simulink model "dual_motor"  (R2020a)
settings: Solver=FixedStepDiscrete  StartTime=0.0  StopTime=10.0  RelTol=1e-3  EnableMultiTasking=on
libraries: REG_Lib x6, TIMERS_Lib x5, GPIO_Lib x3, simulink x2, STM32_Config_Lib x1, USART_Lib x1
settings Model: Creator=Gang  LastModifiedBy=tuziz
settings DataIOCC: LimitDataPoints=on  SaveFormat=Array  ReturnWorkspaceOutputs=off
settings OptimizationCC: DefaultParameterBehavior=Inlined  DefaultUnderspecifiedDataType=single  LifeSpan=1  EfficientTunableParamExpr=on
settings DebuggingCC: UnderspecifiedInitializationDetection=Classic  MergeDetectMultiDrivingBlocksExec=none  InheritedTsInSrcMsg=none  UniqueDataStoreMsg=error  AllowSymbolicDim=off  StrictBusMsg=ErrorOnBusTreatedAsVector  SFUnexpectedBacktrackingDiag=warning  SFNoUnconditionalDefaultTransitionDiag=warning  SFUndirectedBroadcastEventsDiag=error  SFExecutionAtInitializationDiag=none  ArithmeticOperatorsInVariantConditions=warning
settings HardwareCC: ProdBitPerPointer=32  ProdBitPerSizeT=32  ProdBitPerPtrDiffT=32  ProdLargestAtomicInteger=Integer  ProdWordSize=32  ProdHWDeviceType=STMicroelectronics->STM32 32-bit Cortex-M
settings ModelReferenceCC: PropagateSignalLabelsOutOfModel=off
settings SFSimCC: SimUseLocalCustomCode=off  CompileTimeRecursionLimit=0  EnableRuntimeRecursion=off  MATLABDynamicMemAlloc=off  CustomCodeUndefinedFunction=UseInterfaceOnly
settings RTWCC: Description=stm32 (Embedded Target)  SystemTargetFile=stm32.tlc  TemplateMakefile=stm32.tmf  GenerateReport=on  RTWUseLocalCustomCode=off
settings CodeAppCC: IgnoreCustomStorageClasses=off  CustomSymbolStrType=$N$R$M  SimulinkBlockComments=off
settings STFCustomTargetCC: TargetLangStandard=C99 (ISO)  ParMdlRefBuildCompliant=on  IncludeMdlTerminateFcn=off  CombineOutputUpdateFcns=on  ERTCustomFileBanners=on  SupportComplex=off  SupportContinuousTime=off  SupportNonInlinedSFcns=off  RemoveResetFunc=on  ParenthesesLevel=Maximum  CastingMode=Standards  MATLABClassNameForMDSCustomization=Simulink.SoftwareTarget.ERTCustomization  SystemTargetFile=stm32.tlc
settings ERTTargetCC: TargetLangStandard=C99 (ISO)  MultiwordLength=2048  CompOptLevelCompliant=off  ConcurrentExecutionCompliant=off  IncludeMdlTerminateFcn=off  SupportComplex=off  ParenthesesLevel=Maximum  CastingMode=Standards  ModelStepFunctionPrototypeControlCompliant=off  CPPClassGenCompliant=off  UseToolchainInfoCompliant=off  ERTSrcFileBannerTemplate=sourceFileTemplate.cgt  ERTHdrFileBannerTemplate=sourceFileTemplate.cgt  ERTDataSrcFileTemplate=sourceFileTemplate.cgt  ERTDataHdrFileTemplate=sourceFileTemplate.cgt  ERTCustomFileTemplate=customRoutineProcess.tlc  ConvertIfToSwitch=off  SuppressUnreachableDefaultCases=off  EnableSignedLeftShifts=off  EnableSignedRightShifts=off
settings ConfigComp: CovMetricSettings=dw  CovHtmlReporting=on  CovSaveCumulativeToWorkspaceVar=on  CovSaveSingleToWorkspaceVar=on  CovExternalEMLEnable=off  CovSFcnEnable=off

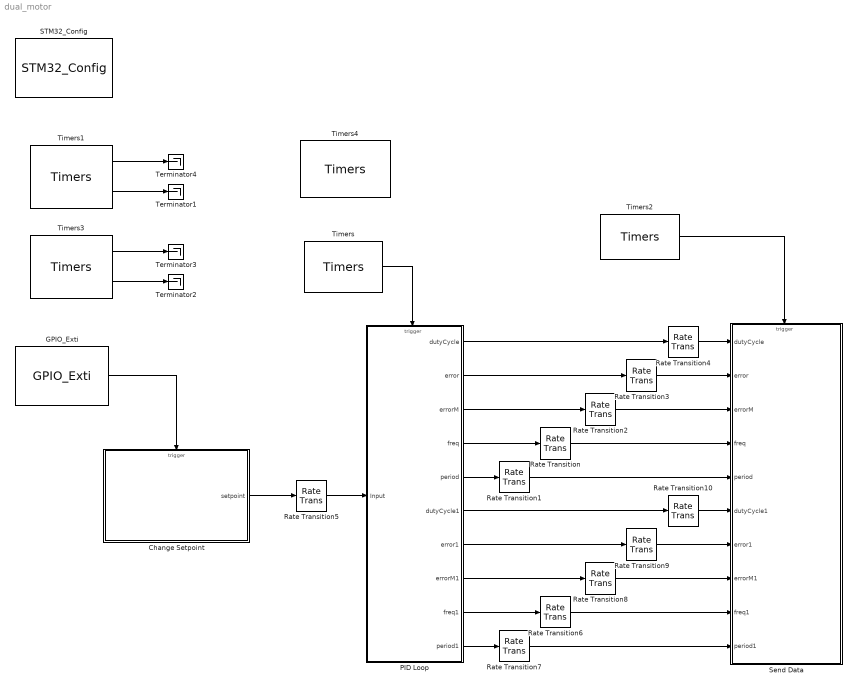
== system dual_motor ==
  Change Setpoint : Subsystem  TreatAsAtomicUnit=on
  GPIO_Exti : GPIO_Lib/GPIO_Exti  Port_name=GPIOA  Pin_0=on  Pin_1=off  Pin_2=off  Pin_3=off  Pin_4=off  Pin_5=off  Pin_6=off  Pin_7=off  Pin_8=off  Pin_9=off  Pin_10=off  Pin_11=off  Pin_12=off  Pin_13=off  Pin_14=off  Pin_15=off  PinList=GPIOA0
      settings: SourceProductName=Target Support Package - STM32 Adapter
  PID Loop : Subsystem  TreatAsAtomicUnit=on
  Rate Transition{,1..10} (11 alike) : RateTransition  Deterministic=off
  STM32_Config : STM32_Config_Lib/STM32_Config  Priority=0  Project_Path=.\  Config_File=dual_motor.ioc  MCU_Name=STM32F407VGTx
      settings: SourceProductName=Target Support Package - STM32 Adapter
  Send Data : Subsystem  TreatAsAtomicUnit=on
  Terminator{1..4} (4 alike) : Terminator
  Timers : TIMERS_Lib/Timers  currentTIM=TIM6  TIM_Name=TIM6  sysUsingTimer=off  TIM_APBClock=84000000  TIM_Set_Clk=off  TIM_Prescaler=8400-1  TIM_Clock=10000.00  Variable_frequency=off  TIM_Set_OutFreq=off  TIM_ARR=10  Output_frequency=1000.00  Repetition_counter=0  TIM_Mode=Up  TIM_DMA=none  TIM_IRQ=off  TIM_IRQ_ONLY=on  TIM_UP=on  TIM_TRG=off  TIM_COM=off  TIM_BRK=off  NbTIM=5  CH1_enable=off  CH1N_enable=off  CH1_type=Unknown  CH1_DMA=off  CH1_int=off  CH1_edge=Rising  CH1_div=1  CH1_variable_duty=off  CH1_set_pulse=off  CH1_output_duty=0.00  CH1_pulse=0  CH2_enable=off  CH2N_enable=off  CH2_type=Unknown  CH2_DMA=off  CH2_int=off  CH2_edge=Rising  CH2_div=1  CH2_variable_duty=off  CH2_set_pulse=off  CH2_output_duty=0.00  CH2_pulse=0  CH3_enable=off  CH3N_enable=off  CH3_type=Unknown  CH3_DMA=off  CH3_int=off  CH3_edge=Rising  CH3_div=1  CH3_variable_duty=off  CH3_set_pulse=off  CH3_output_duty=0.00  CH3_pulse=0  CH4_enable=off  CH4N_enable=off  CH4_type=Unknown  CH4_DMA=off  CH4_int=off  CH4_edge=Rising  CH4_div=1  CH4_variable_duty=off  CH4_set_pulse=off  CH4_output_duty=0.00  CH4_pulse=0
      settings: SourceProductName=Target Support Package - STM32 Adapter
  Timers1 : TIMERS_Lib/Timers  currentTIM=TIM3  TIM_Name=TIM3  sysUsingTimer=off  TIM_APBClock=84000000  TIM_Set_Clk=off  TIM_Prescaler=840-1  TIM_Clock=100000.00  Variable_frequency=off  TIM_Set_OutFreq=off  TIM_ARR=2000  Output_frequency=50.00  Repetition_counter=0  TIM_Mode=Up  TIM_DMA=none  TIM_IRQ=off  TIM_IRQ_ONLY=off  TIM_UP=off  TIM_TRG=off  TIM_COM=off  TIM_BRK=off  NbTIM=5  CH1_enable=on  CH1N_enable=off  CH1_type=Input_Capture  CH1_DMA=off  CH1_int=on  CH1_edge=Rising  CH1_div=1  CH1_variable_duty=off  CH1_set_pulse=off  CH1_output_duty=0.00  CH1_pulse=0  CH2_enable=off  CH2N_enable=off  CH2_type=Input_Capture  CH2_DMA=off  CH2_int=off  CH2_edge=Rising  CH2_div=1  CH2_variable_duty=off  CH2_set_pulse=off  CH2_output_duty=0.00  CH2_pulse=0  CH3_enable=off  CH3N_enable=off  CH3_type=Unknown  CH3_DMA=off  CH3_int=off  CH3_edge=Rising  CH3_div=1  CH3_variable_duty=off  CH3_set_pulse=off  CH3_output_duty=0.00  CH3_pulse=0  CH4_enable=off  CH4N_enable=off  CH4_type=Unknown  CH4_DMA=off  CH4_int=off  CH4_edge=Rising  CH4_div=1  CH4_variable_duty=off  CH4_set_pulse=off  CH4_output_duty=0.00  CH4_pulse=0
      settings: SourceProductName=Target Support Package - STM32 Adapter
  Timers2 : TIMERS_Lib/Timers  currentTIM=TIM7  TIM_Name=TIM7  sysUsingTimer=off  TIM_APBClock=84000000  TIM_Set_Clk=off  TIM_Prescaler=840-1  TIM_Clock=100000.00  Variable_frequency=off  TIM_Set_OutFreq=off  TIM_ARR=1000  Output_frequency=100.00  Repetition_counter=0  TIM_Mode=Up  TIM_DMA=none  TIM_IRQ=off  TIM_IRQ_ONLY=on  TIM_UP=on  TIM_TRG=off  TIM_COM=off  TIM_BRK=off  NbTIM=5  CH1_enable=off  CH1N_enable=off  CH1_type=Unknown  CH1_DMA=off  CH1_int=off  CH1_edge=Rising  CH1_div=1  CH1_variable_duty=off  CH1_set_pulse=off  CH1_output_duty=0.00  CH1_pulse=0  CH2_enable=off  CH2N_enable=off  CH2_type=Unknown  CH2_DMA=off  CH2_int=off  CH2_edge=Rising  CH2_div=1  CH2_variable_duty=off  CH2_set_pulse=off  CH2_output_duty=0.00  CH2_pulse=0  CH3_enable=off  CH3N_enable=off  CH3_type=Unknown  CH3_DMA=off  CH3_int=off  CH3_edge=Rising  CH3_div=1  CH3_variable_duty=off  CH3_set_pulse=off  CH3_output_duty=0.00  CH3_pulse=0  CH4_enable=off  CH4N_enable=off  CH4_type=Unknown  CH4_DMA=off  CH4_int=off  CH4_edge=Rising  CH4_div=1  CH4_variable_duty=off  CH4_set_pulse=off  CH4_output_duty=0.00  CH4_pulse=0
      settings: SourceProductName=Target Support Package - STM32 Adapter
  Timers3 : TIMERS_Lib/Timers  currentTIM=TIM4  TIM_Name=TIM4  sysUsingTimer=off  TIM_APBClock=84000000  TIM_Set_Clk=off  TIM_Prescaler=840-1  TIM_Clock=100000.00  Variable_frequency=off  TIM_Set_OutFreq=off  TIM_ARR=2000  Output_frequency=50.00  Repetition_counter=0  TIM_Mode=Up  TIM_DMA=none  TIM_IRQ=off  TIM_IRQ_ONLY=off  TIM_UP=off  TIM_TRG=off  TIM_COM=off  TIM_BRK=off  NbTIM=5  CH1_enable=on  CH1N_enable=off  CH1_type=Input_Capture  CH1_DMA=off  CH1_int=on  CH1_edge=Rising  CH1_div=1  CH1_variable_duty=off  CH1_set_pulse=off  CH1_output_duty=0.00  CH1_pulse=0  CH2_enable=off  CH2N_enable=off  CH2_type=Unknown  CH2_DMA=off  CH2_int=off  CH2_edge=Rising  CH2_div=1  CH2_variable_duty=off  CH2_set_pulse=off  CH2_output_duty=0.00  CH2_pulse=0  CH3_enable=off  CH3N_enable=off  CH3_type=Unknown  CH3_DMA=off  CH3_int=off  CH3_edge=Rising  CH3_div=1  CH3_variable_duty=off  CH3_set_pulse=off  CH3_output_duty=0.00  CH3_pulse=0  CH4_enable=off  CH4N_enable=off  CH4_type=Unknown  CH4_DMA=off  CH4_int=off  CH4_edge=Rising  CH4_div=1  CH4_variable_duty=off  CH4_set_pulse=off  CH4_output_duty=0.00  CH4_pulse=0
      settings: SourceProductName=Target Support Package - STM32 Adapter
  Timers4 : TIMERS_Lib/Timers  currentTIM=TIM9  TIM_Name=TIM9  sysUsingTimer=off  TIM_APBClock=168000000  TIM_Set_Clk=off  TIM_Prescaler=3359  TIM_Clock=50000.00  Variable_frequency=off  TIM_Set_OutFreq=off  TIM_ARR=100  Output_frequency=500.00  Repetition_counter=0  TIM_Mode=Up  TIM_DMA=none  TIM_IRQ=off  TIM_IRQ_ONLY=off  TIM_UP=off  TIM_TRG=off  TIM_COM=off  TIM_BRK=off  NbTIM=5  CH1_enable=on  CH1N_enable=off  CH1_type=Output_PWM  CH1_DMA=off  CH1_int=off  CH1_edge=Rising  CH1_div=1  CH1_variable_duty=off  CH1_set_pulse=off  CH1_output_duty=0.00  CH1_pulse=0  CH2_enable=on  CH2N_enable=off  CH2_type=Output_PWM  CH2_DMA=off  CH2_int=off  CH2_edge=Rising  CH2_div=1  CH2_variable_duty=off  CH2_set_pulse=off  CH2_output_duty=0.00  CH2_pulse=0  CH3_enable=off  CH3N_enable=off  CH3_type=Unknown  CH3_DMA=off  CH3_int=off  CH3_edge=Rising  CH3_div=1  CH3_variable_duty=off  CH3_set_pulse=off  CH3_output_duty=0.00  CH3_pulse=0  CH4_enable=off  CH4N_enable=off  CH4_type=Unknown  CH4_DMA=off  CH4_int=off  CH4_edge=Rising  CH4_div=1  CH4_variable_duty=off  CH4_set_pulse=off  CH4_output_duty=0.00  CH4_pulse=0
      settings: SourceProductName=Target Support Package - STM32 Adapter
  wires:
  Timers2/1 -> Send Data/Trigger
  Timers1/2 -> Terminator1/1
  PID Loop/4(freq) -> Rate Transition/1
  PID Loop/5(period) -> Rate Transition1/1
  Rate Transition/1 -> Send Data/4(freq)
  Rate Transition1/1 -> Send Data/5(period)
  Rate Transition2/1 -> Send Data/3(errorM)
  PID Loop/3(errorM) -> Rate Transition2/1
  PID Loop/2(error) -> Rate Transition3/1
  Rate Transition3/1 -> Send Data/2(error)
  Rate Transition4/1 -> Send Data/1(dutyCycle)
  PID Loop/1(dutyCycle) -> Rate Transition4/1
  GPIO_Exti/1 -> Change Setpoint/Trigger
  Change Setpoint/1(setpoint) -> Rate Transition5/1
  Rate Transition5/1 -> PID Loop/1(Input)
  PID Loop/6(dutyCycle1) -> Rate Transition10/1
  Rate Transition9/1 -> Send Data/7(error1)
  PID Loop/7(error1) -> Rate Transition9/1
  PID Loop/8(errorM1) -> Rate Transition8/1
  Rate Transition8/1 -> Send Data/8(errorM1)
  Rate Transition7/1 -> Send Data/10(period1)
  Rate Transition6/1 -> Send Data/9(freq1)
  PID Loop/9(freq1) -> Rate Transition6/1
  PID Loop/10(period1) -> Rate Transition7/1
  Rate Transition10/1 -> Send Data/6(dutyCycle1)
  Timers3/1 -> Terminator3/1
  Timers3/2 -> Terminator2/1
  Timers1/1 -> Terminator4/1
  Timers/1 -> PID Loop/Trigger

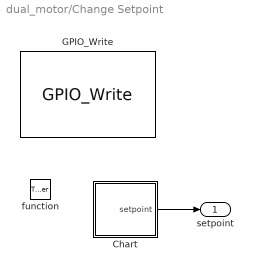
== system dual_motor/Change Setpoint ==
  function : TriggerPort  TriggerType=function-call  VariantControl=Variant  OutputDataType=int8
  Chart : Stateflow chart  TreatAsAtomicUnit=on
  GPIO_Write : GPIO_Lib/GPIO_Write  Port_name=GPIOD  Pin0=off  Toggle_Pin0=off  Pin1=off  Toggle_Pin1=off  Pin2=off  Toggle_Pin2=off  Pin3=off  Toggle_Pin3=off  Pin4=off  Toggle_Pin4=off  Pin5=off  Toggle_Pin5=off  Pin6=off  Toggle_Pin6=off  Pin7=off  Toggle_Pin7=off  Pin8=off  Toggle_Pin8=off  Pin9=off  Toggle_Pin9=off  Pin10=off  Toggle_Pin10=off  Pin11=off  Toggle_Pin11=off  Pin12=off  Toggle_Pin12=off  Pin13=off  Toggle_Pin13=off  Pin14=on  Toggle_Pin14=on  Pin15=off  Toggle_Pin15=off  PinList="GPIOD12  13  14  15"
      settings: SourceProductName=Target Support Package - STM32 Adapter
  setpoint : Outport
  wires:
  Chart/1(setpoint) -> setpoint/1

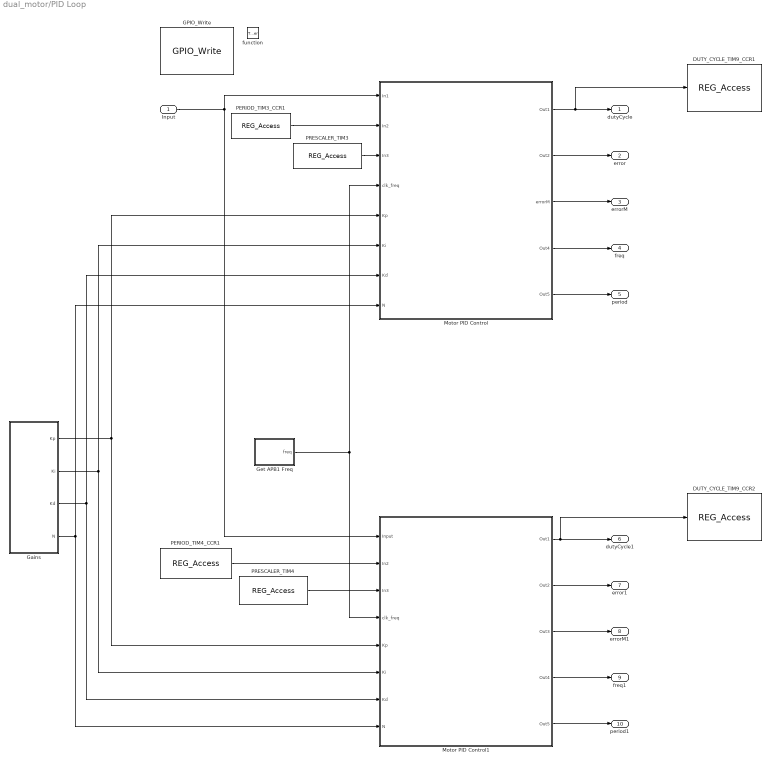
== system dual_motor/PID Loop ==
  Input : Inport
  function : TriggerPort  TriggerType=function-call  VariantControl=Variant
  DUTY_CYCLE_TIM9_CCR1 : REG_Lib/REG_Access  Peripheral=TIM9  RegName=CCR1  RegRead=off  RegWrite=on  RegValueIn=on  RegEqual=on  RegAnd=off  RegOr=off  RegComplement=off  currentPeriph=TIM9
      settings: SourceProductName=Target Support Package - STM32 Adapter
  DUTY_CYCLE_TIM9_CCR2 : REG_Lib/REG_Access  Peripheral=TIM9  RegName=CCR2  RegRead=off  RegWrite=on  RegValueIn=on  RegEqual=on  RegAnd=off  RegOr=off  RegComplement=off  currentPeriph=TIM9
      settings: SourceProductName=Target Support Package - STM32 Adapter
  GPIO_Write : GPIO_Lib/GPIO_Write  Port_name=GPIOD  Pin0=off  Toggle_Pin0=off  Pin1=off  Toggle_Pin1=off  Pin2=off  Toggle_Pin2=off  Pin3=off  Toggle_Pin3=off  Pin4=off  Toggle_Pin4=off  Pin5=off  Toggle_Pin5=off  Pin6=off  Toggle_Pin6=off  Pin7=off  Toggle_Pin7=off  Pin8=off  Toggle_Pin8=off  Pin9=off  Toggle_Pin9=off  Pin10=off  Toggle_Pin10=off  Pin11=off  Toggle_Pin11=off  Pin12=off  Toggle_Pin12=off  Pin13=on  Toggle_Pin13=on  Pin14=off  Toggle_Pin14=off  Pin15=off  Toggle_Pin15=off  PinList="GPIOD12  13  14  15"
      settings: SourceProductName=Target Support Package - STM32 Adapter
  Gains : MATLAB Function  TreatAsAtomicUnit=on
  Get APB1 Freq : MATLAB Function  TreatAsAtomicUnit=on
  Motor PID Control : Subsystem
  Motor PID Control1 : Subsystem
  PERIOD_TIM3_CCR1 : REG_Lib/REG_Access  Peripheral=TIM3  RegName=CCR1  RegRead=on  RegWrite=off  RegValueIn=off  RegEqual=on  RegAnd=off  RegOr=off  RegComplement=off  currentPeriph=TIM3
      settings: SourceProductName=Target Support Package - STM32 Adapter
  PERIOD_TIM4_CCR1 : REG_Lib/REG_Access  Peripheral=TIM4  RegName=CCR1  RegRead=on  RegWrite=off  RegValueIn=off  RegEqual=on  RegAnd=off  RegOr=off  RegComplement=off  currentPeriph=TIM4
      settings: SourceProductName=Target Support Package - STM32 Adapter
  PRESCALER_TIM3 : REG_Lib/REG_Access  Peripheral=TIM3  RegName=PSC  RegRead=on  RegWrite=off  RegValueIn=off  RegEqual=on  RegAnd=off  RegOr=off  RegComplement=off  currentPeriph=TIM3
      settings: SourceProductName=Target Support Package - STM32 Adapter
  PRESCALER_TIM4 : REG_Lib/REG_Access  Peripheral=TIM4  RegName=PSC  RegRead=on  RegWrite=off  RegValueIn=off  RegEqual=on  RegAnd=off  RegOr=off  RegComplement=off  currentPeriph=TIM4
      settings: SourceProductName=Target Support Package - STM32 Adapter
  dutyCycle : Outport
  error : Outport  Port=2
  errorM : Outport  Port=3
  freq : Outport  Port=4
  period : Outport  Port=5
  dutyCycle1 : Outport  Port=6
  error1 : Outport  Port=7
  errorM1 : Outport  Port=8
  freq1 : Outport  Port=9
  period1 : Outport  Port=10
  wires:
  Motor PID Control/1(Out1) -> DUTY_CYCLE_TIM9_CCR1/1, dutyCycle/1
  PERIOD_TIM3_CCR1/1 -> Motor PID Control/2(In2)
  Motor PID Control/2(Out2) -> error/1
  Motor PID Control/4(Out4) -> freq/1
  Motor PID Control/5(Out5) -> period/1
  Input/1 -> Motor PID Control1/1(Input), Motor PID Control/1(In1)
  Motor PID Control1/5(Out5) -> period1/1
  Motor PID Control1/4(Out4) -> freq1/1
  Motor PID Control1/3(Out3) -> errorM1/1
  Motor PID Control1/2(Out2) -> error1/1
  PERIOD_TIM4_CCR1/1 -> Motor PID Control1/2(In2)
  Motor PID Control1/1(Out1) -> DUTY_CYCLE_TIM9_CCR2/1, dutyCycle1/1
  Get APB1 Freq/1(freq) -> Motor PID Control/4(clk_freq), Motor PID Control1/4(clk_freq)
  PRESCALER_TIM3/1 -> Motor PID Control/3(In3)
  PRESCALER_TIM4/1 -> Motor PID Control1/3(In3)
  Motor PID Control/3(errorM) -> errorM/1
  Gains/1(Kp) -> Motor PID Control/5(Kp), Motor PID Control1/5(Kp)
  Gains/2(Ki) -> Motor PID Control/6(Ki), Motor PID Control1/6(Ki)
  Gains/3(Kd) -> Motor PID Control/7(Kd), Motor PID Control1/7(Kd)
  Gains/4(N) -> Motor PID Control/8(N), Motor PID Control1/8(N)

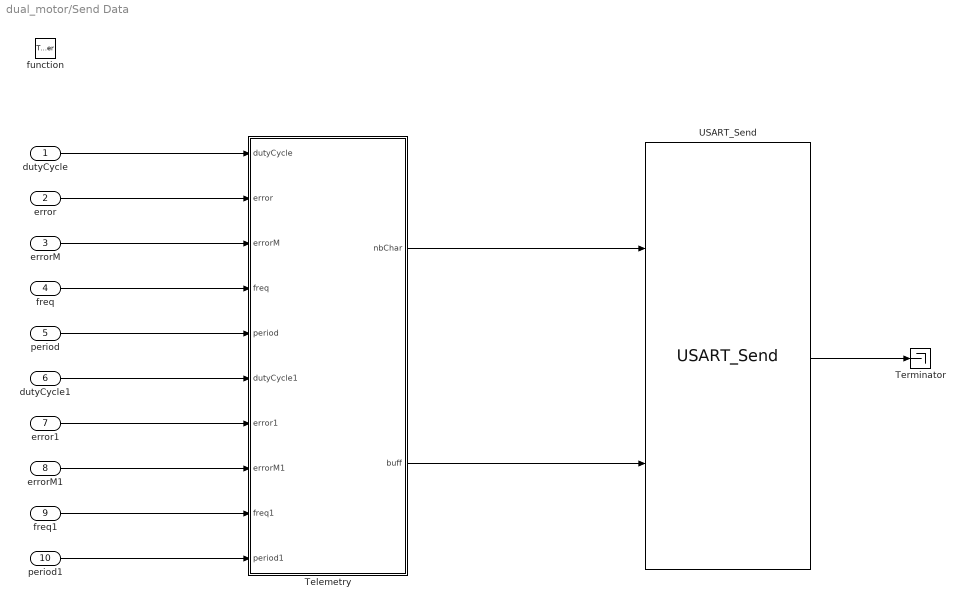
== system dual_motor/Send Data ==
  dutyCycle : Inport
  error : Inport  Port=2
  errorM : Inport  Port=3
  freq : Inport  Port=4
  period : Inport  Port=5
  dutyCycle1 : Inport  Port=6
  error1 : Inport  Port=7
  errorM1 : Inport  Port=8
  freq1 : Inport  Port=9
  period1 : Inport  Port=10
  function : TriggerPort  TriggerType=function-call  VariantControl=Variant
  Telemetry : MATLAB Function  TreatAsAtomicUnit=on
  Terminator : Terminator
  USART_Send : USART_Lib/USART_Send  USART_name=USART3  Buff_size=512  nbUsart=1  usartMode=Asynchronous  usartDma_Rx=off  usartDma_Tx=off  usartIt=off
      settings: SourceProductName=Target Support Package - STM32 Adapter
  wires:
  USART_Send/1 -> Terminator/1
  period/1 -> Telemetry/5(period)
  freq/1 -> Telemetry/4(freq)
  dutyCycle/1 -> Telemetry/1(dutyCycle)
  error/1 -> Telemetry/2(error)
  errorM/1 -> Telemetry/3(errorM)
  Telemetry/1(nbChar) -> USART_Send/1
  Telemetry/2(buff) -> USART_Send/2
  period1/1 -> Telemetry/10(period1)
  freq1/1 -> Telemetry/9(freq1)
  dutyCycle1/1 -> Telemetry/6(dutyCycle1)
  error1/1 -> Telemetry/7(error1)
  errorM1/1 -> Telemetry/8(errorM1)

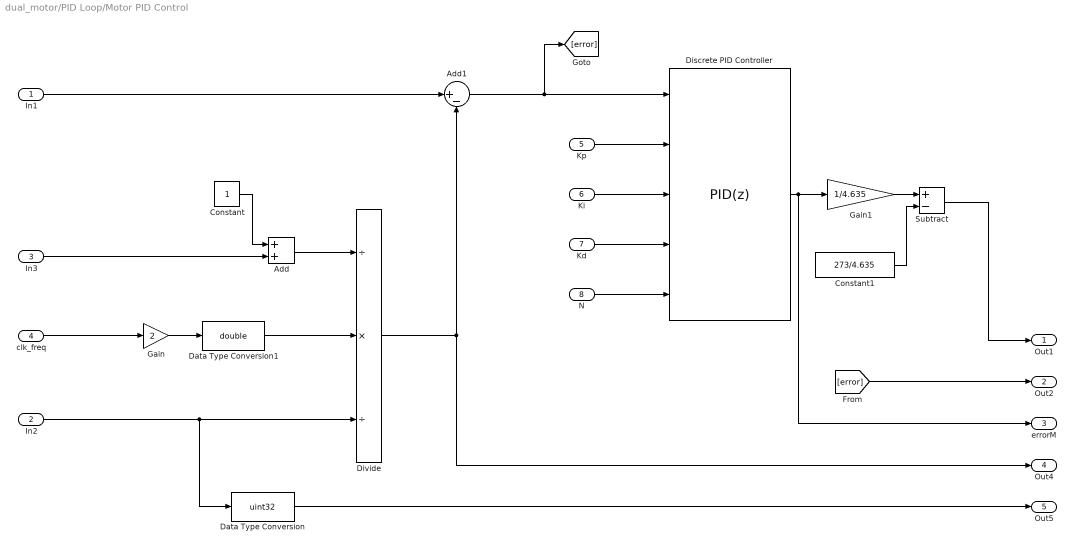
== system dual_motor/PID Loop/Motor PID Control ==
  In1 : Inport
  In2 : Inport  Port=2
  In3 : Inport  Port=3
  clk_freq : Inport  Port=4
  Kp : Inport  Port=5
  Ki : Inport  Port=6
  Kd : Inport  Port=7
  N : Inport  Port=8
  Add : Sum  OutDataTypeStr=double
  Add1 : Sum  Inputs=|+-  OutDataTypeStr=double
  Constant : Constant  OutDataTypeStr=double
  Constant1 : Constant  Value=273/4.635
  Data Type Conversion : DataTypeConversion  OutDataTypeStr=uint32
  Data Type Conversion1 : DataTypeConversion  OutDataTypeStr=double
  Discrete PID Controller : simulink/Continuous/PID Controller  Controller=PID  Form=Parallel  TimeDomain=Discrete-time  UseExternalTs=off  SampleTime=-1  IntegratorMethod=Forward Euler  FilterMethod=Forward Euler  ControllerParametersSource=external  P=50.0  I=5  D=.5  UseFilter=on  N=100  TunerSelectOption=Transfer Function Based (PID Tuner App)  InitialConditionSource=internal  InitialConditionForIntegrator=0  InitialConditionForFilter=0  DifferentiatorICPrevScaledInput=0  ExternalReset=none  TrackingMode=off  Kt=1  LimitOutput=on  UpperSaturationLimit=700  LowerSaturationLimit=273  LinearizeAsGain=off  AntiWindupMode=clamping  Kb=1  POutMin=[]  POutMax=[]  IOutMin=[]  IOutMax=[]  DOutMin=[]  DOutMax=[]  NOutMin=[]  NOutMax=[]  SumOutMin=[]  SumOutMax=[]  SaturationOutMin=[]  SaturationOutMax=[]  PParamMin=[]  PParamMax=[]  IParamMin=[]  IParamMax=[]  DParamMin=[]  DParamMax=[]  NParamMin=[]  NParamMax=[]  KbParamMin=[]  KbParamMax=[]  KtParamMin=[]  KtParamMax=[]  KbOutMin=[]  KbOutMax=[]  KtOutMin=[]  KtOutMax=[]  IntegratorOutMin=[]  IntegratorOutMax=[]  FilterOutMin=[]  FilterOutMax=[]  SumI1OutMin=[]  SumI1OutMax=[]  SumI2OutMin=[]  SumI2OutMax=[]  SumI3OutMin=[]  SumI3OutMax=[]  SumI4OutMin=[]  SumI4OutMax=[]  SumDOutMin=[]  SumDOutMax=[]  DifferentiatorOutMin=[]  DifferentiatorOutMax=[]  FilterDiffOutCoefMin=[]  FilterDiffOutCoefMax=[]  ReciprocalOutMin=[]  ReciprocalOutMax=[]  SumDenOutMin=[]  SumDenOutMax=[]  SumNumOutMin=[]  SumNumOutMax=[]  DivideOutMin=[]  DivideOutMax=[]  UdiffTsProdOutMin=[]  UdiffTsProdOutMax=[]  NTsProdOutMin=[]  NTsProdOutMax=[]  UintegralTsProdOutMin=[]  UintegralTsProdOutMax=[]  UngainTsProdOutMin=[]  UngainTsProdOutMax=[]  IntegratorContinuousStateAttributes=''  IntegratorStateMustResolveToSignalObject=off  IntegratorRTWStateStorageClass=Auto  FilterContinuousStateAttributes=''  FilterStateMustResolveToSignalObject=off  FilterRTWStateStorageClass=Auto  ParallelPVariant=ExternalParameters  IdealPVariant=Disabled  IVariant=ExternalParameters  DVariant=ExternalParameters  IntegratorVariant=Discrete  SatVariant=Enabled  AWVariant=DiscClampingParallel  PCopyVariant=Disabled  TRVariant=Disabled  FdbkBlocksVariant=Forward  IdealPFdbkVariant=Disabled  SatFdbkVariant=Disabled  DerivativeFilterVariant=ForwardEulerFilter  NVariant=ExternalParameters  NCopyVariant=Disabled  FilterICVariant=InternalICsFilter  IntegratorICVariant=InternalICs  ExternalResetVariant=Disabled  TRSumVariant=Passthrough  SumFdbkVariant=Disabled  SumVariant=Sum_PID  TsampFilterVariant=InternalTs  TsampNgainVariant=Passthrough  TsampIntegralVariant=Passthrough
  Divide : Product  Inputs=/*/  OutDataTypeStr=double
  Gain : Gain  Gain=2  ParamDataTypeStr=double  OutDataTypeStr=double
  Gain1 : Gain  Gain=1/4.635  OutDataTypeStr=double
  Subtract : Sum  Inputs=+-
  Out1 : Outport
  Out2 : Outport  Port=2
  errorM : Outport  Port=3
  Out4 : Outport  Port=4
  Out5 : Outport  Port=5
  wires:
  In3/1 -> Add/2
  Data Type Conversion/1 -> Out5/1
  Add1/1 -> [error], Discrete PID Controller/1
  Constant/1 -> Add/1
  In2/1 -> Data Type Conversion/1, Divide/3
  Add/1 -> Divide/1
  Divide/1 -> Out4/1, Add1/2
  Discrete PID Controller/1 -> Gain1/1, errorM/1
  Kd/1 -> Discrete PID Controller/4
  clk_freq/1 -> Gain/1
  Kp/1 -> Discrete PID Controller/2
  Gain/1 -> Data Type Conversion1/1
  Ki/1 -> Discrete PID Controller/3
  [error] -> Out2/1
  Data Type Conversion1/1 -> Divide/2
  N/1 -> Discrete PID Controller/5
  In1/1 -> Add1/1
  Gain1/1 -> Subtract/1
  Subtract/1 -> Out1/1
  Constant1/1 -> Subtract/2

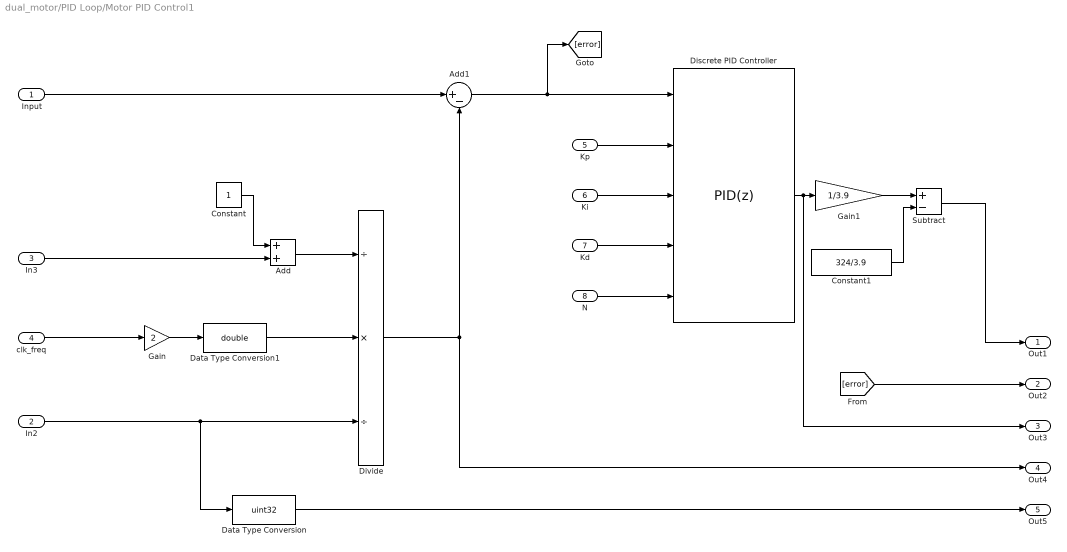
== system dual_motor/PID Loop/Motor PID Control1 ==
  Input : Inport
  In2 : Inport  Port=2
  In3 : Inport  Port=3
  clk_freq : Inport  Port=4
  Kp : Inport  Port=5
  Ki : Inport  Port=6
  Kd : Inport  Port=7
  N : Inport  Port=8
  Add : Sum  OutDataTypeStr=double
  Add1 : Sum  Inputs=|+-  OutDataTypeStr=double
  Constant : Constant  OutDataTypeStr=double
  Constant1 : Constant  Value=324/3.9
  Data Type Conversion : DataTypeConversion  OutDataTypeStr=uint32
  Data Type Conversion1 : DataTypeConversion  OutDataTypeStr=double
  Discrete PID Controller : simulink/Continuous/PID Controller  Controller=PID  Form=Parallel  TimeDomain=Discrete-time  UseExternalTs=off  SampleTime=-1  IntegratorMethod=Forward Euler  FilterMethod=Forward Euler  ControllerParametersSource=external  P=50.0  I=5  D=.5  UseFilter=on  N=100  TunerSelectOption=Transfer Function Based (PID Tuner App)  InitialConditionSource=internal  InitialConditionForIntegrator=0  InitialConditionForFilter=0  DifferentiatorICPrevScaledInput=0  ExternalReset=none  TrackingMode=off  Kt=1  LimitOutput=on  UpperSaturationLimit=700  LowerSaturationLimit=324  LinearizeAsGain=off  AntiWindupMode=clamping  Kb=1  POutMin=[]  POutMax=[]  IOutMin=[]  IOutMax=[]  DOutMin=[]  DOutMax=[]  NOutMin=[]  NOutMax=[]  SumOutMin=[]  SumOutMax=[]  SaturationOutMin=[]  SaturationOutMax=[]  PParamMin=[]  PParamMax=[]  IParamMin=[]  IParamMax=[]  DParamMin=[]  DParamMax=[]  NParamMin=[]  NParamMax=[]  KbParamMin=[]  KbParamMax=[]  KtParamMin=[]  KtParamMax=[]  KbOutMin=[]  KbOutMax=[]  KtOutMin=[]  KtOutMax=[]  IntegratorOutMin=[]  IntegratorOutMax=[]  FilterOutMin=[]  FilterOutMax=[]  SumI1OutMin=[]  SumI1OutMax=[]  SumI2OutMin=[]  SumI2OutMax=[]  SumI3OutMin=[]  SumI3OutMax=[]  SumI4OutMin=[]  SumI4OutMax=[]  SumDOutMin=[]  SumDOutMax=[]  DifferentiatorOutMin=[]  DifferentiatorOutMax=[]  FilterDiffOutCoefMin=[]  FilterDiffOutCoefMax=[]  ReciprocalOutMin=[]  ReciprocalOutMax=[]  SumDenOutMin=[]  SumDenOutMax=[]  SumNumOutMin=[]  SumNumOutMax=[]  DivideOutMin=[]  DivideOutMax=[]  UdiffTsProdOutMin=[]  UdiffTsProdOutMax=[]  NTsProdOutMin=[]  NTsProdOutMax=[]  UintegralTsProdOutMin=[]  UintegralTsProdOutMax=[]  UngainTsProdOutMin=[]  UngainTsProdOutMax=[]  IntegratorContinuousStateAttributes=''  IntegratorStateMustResolveToSignalObject=off  IntegratorRTWStateStorageClass=Auto  FilterContinuousStateAttributes=''  FilterStateMustResolveToSignalObject=off  FilterRTWStateStorageClass=Auto  ParallelPVariant=ExternalParameters  IdealPVariant=Disabled  IVariant=ExternalParameters  DVariant=ExternalParameters  IntegratorVariant=Discrete  SatVariant=Enabled  AWVariant=DiscClampingParallel  PCopyVariant=Disabled  TRVariant=Disabled  FdbkBlocksVariant=Forward  IdealPFdbkVariant=Disabled  SatFdbkVariant=Disabled  DerivativeFilterVariant=ForwardEulerFilter  NVariant=ExternalParameters  NCopyVariant=Disabled  FilterICVariant=InternalICsFilter  IntegratorICVariant=InternalICs  ExternalResetVariant=Disabled  TRSumVariant=Passthrough  SumFdbkVariant=Disabled  SumVariant=Sum_PID  TsampFilterVariant=InternalTs  TsampNgainVariant=Passthrough  TsampIntegralVariant=Passthrough
  Divide : Product  Inputs=/*/  OutDataTypeStr=double
  Gain : Gain  Gain=2  ParamDataTypeStr=double  OutDataTypeStr=double
  Gain1 : Gain  Gain=1/3.9  OutDataTypeStr=double
  Subtract : Sum  Inputs=+-
  Out1 : Outport
  Out2 : Outport  Port=2
  Out3 : Outport  Port=3
  Out4 : Outport  Port=4
  Out5 : Outport  Port=5
  wires:
  Input/1 -> Add1/1
  N/1 -> Discrete PID Controller/5
  Data Type Conversion1/1 -> Divide/2
  [error] -> Out2/1
  Ki/1 -> Discrete PID Controller/3
  Gain/1 -> Data Type Conversion1/1
  Kp/1 -> Discrete PID Controller/2
  clk_freq/1 -> Gain/1
  Kd/1 -> Discrete PID Controller/4
  Discrete PID Controller/1 -> Gain1/1, Out3/1
  Divide/1 -> Add1/2, Out4/1
  Add/1 -> Divide/1
  In2/1 -> Divide/3, Data Type Conversion/1
  Constant/1 -> Add/1
  Add1/1 -> Discrete PID Controller/1, [error]
  Data Type Conversion/1 -> Out5/1
  In3/1 -> Add/2
  Subtract/1 -> Out1/1
  Constant1/1 -> Subtract/2
  Gain1/1 -> Subtract/1

== matlab function dual_motor/Send Data/Telemetry ==
  data: dutyCycle input; error input; errorM input; freq input; nbChar output uint16 size=1; buff output uint32 size=1; period input; dutyCycle1 input; error1 input; errorM1 input; freq1 input; period1 input
function [nbChar, buff] = convert(dutyCycle,error,errorM,freq,period,dutyCycle1,error1,errorM1,freq1,period1)
if coder.target('Sfun')
    % Executing in MATLAB, Buff is null
    buff = uint32(0);
    nbChar = uint16(0);
else
    coder.cinclude('stdio.h');
    coder.cinclude('main.h');
    coder.cinclude('getBuffPtr.h');

    % Executing in the generated code.
    string = char(zeros(1,100));
    stringSize = uint16(size(string,2));
    stringFormat = char(['%u,','%5.2f,','%5.2f,','%5.2f,','%5.2f,','%u,','%5.2f,','%5.2f,','%5.2f,','%5.2f',13,10,0]);
    coder.ceval('snprintf',coder.wref(string),stringSize,coder.rref(stringFormat),period,error,errorM,freq,dutyCycle,period1,error1,errorM1,freq1,dutyCycle1);
    buff = coder.ceval('getBuffPtr',coder.rref(string));
    nbChar = stringSize - 30;
end
end

== matlab function dual_motor/PID Loop/Gains ==
  data: Kp output; Ki output; Kd output; N output
function [Kp,Ki,Kd,N] = fcn()
Kp = 10.0;
Ki = 3.0;
Kd = 40.0;
N = 100.0;
end

== stateflow chart dual_motor/Change Setpoint/Chart ==
  state S1
    setpoint=150.00;
  state S2
    setpoint=300.00;
  state S4
    setpoint=600.00;
  state S3
    setpoint=450.00;
  (default) -> S1
  S1 -> S2
  S4 -> S1
  S2 -> S3
  S3 -> S4
  data: setpoint output

== matlab function dual_motor/PID Loop/Get APB1 Freq ==
  data: freq output
function freq = fcn()
if coder.target('Sfun')
    % Executing in MATLAB, Buff is null
    freq = double(0);
else
    coder.cinclude('stm32f4xx_hal_rcc.h');
    
    % Executing in the generated code.
    freq = coder.ceval('HAL_RCC_GetPCLK1Freq');
end
end
